simulink model "cq3_2019"  (R2024b)
settings: Solver=FixedStepAuto  StartTime=0.0  StopTime=10  FixedStep=0.001  RelTol=1e-3
libraries: simulink x3, Solver_SF x1
settings Model: SnapshotBufferSize=2  SnapshotInterval=1  Creator=user  LastModifiedBy=user

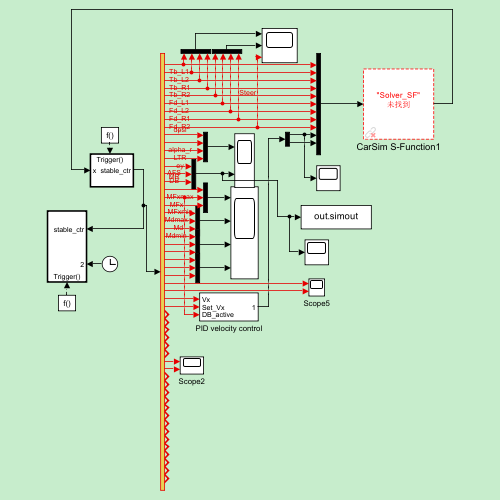
[thumbnail: Simulink's stored preview of the top-level diagram]
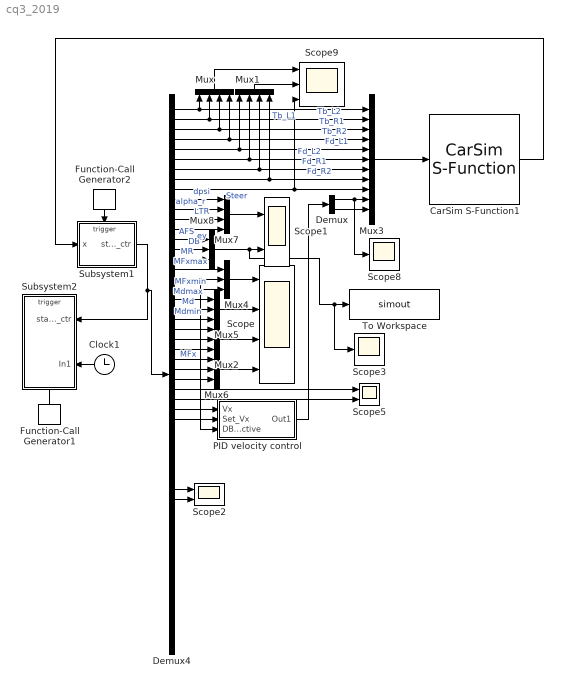
== system cq3_2019 ==
  CarSim S-Function1 : Solver_SF/CarSim S-Function  Priority=1  SIMFILE=simfile.sim
  Clock1 : Clock
  Demux : Demux  Outputs=2
  Demux4 : Demux  Outputs=54
  Function-Call Generator1 : simulink/Ports & Subsystems/Function-Call Generator  sample_time=0.01  numberOfIterations=1  DisallowWideOutput=off
  Function-Call Generator2 : simulink/Ports & Subsystems/Function-Call Generator  sample_time=0.01  numberOfIterations=1  DisallowWideOutput=off
  Mux : Mux
  Mux1 : Mux
  Mux{2,4..6,8} (5 alike) : Mux  Inputs=3
  Mux3 : Mux  Inputs=11
  Mux7 : Mux
  PID velocity control : Subsystem
  Scope : Scope  NumInputPorts=4
  Scope1 : Scope  NumInputPorts=2
  Scope2 : Scope  NumInputPorts=2
  Scope3 : Scope
  Scope5 : Scope  NumInputPorts=2
  Scope8 : Scope
  Scope9 : Scope  NumInputPorts=3
  Subsystem1 : Subsystem
  Subsystem2 : Subsystem
  To Workspace : ToWorkspace  VariableName=simout  SaveFormat=Timeseries  SampleTime=-1
  wires:
  Demux4/4 -> Mux/4, Mux3/4  "Tb_R2"
  Demux4/19 -> Mux4/3  "MFxmin"
  Demux4/26 -> Mux6/1
  Demux4/21 -> Mux5/2  "Md"
  CarSim S-Function1/1 -> Subsystem1/1(x)
  Demux4/3 -> Mux/3, Mux3/3  "Tb_R1"
  Demux4/17 -> Mux4/1  "MFxmax"
  Demux4/18 -> Mux4/2, PID velocity control/3(DB_active)  "MFx"
  Demux4/8 -> Mux1/4, Mux3/8  "Fd_R2"
  Demux4/5 -> Mux1/1, Mux3/5  "Fd_L1"
  Demux4/15 -> Mux8/2  "DB"
  Demux4/27 -> Mux6/2
  Demux4/11 -> Mux7/2  "alpha_r"
  Demux4/20 -> Mux5/1  "Mdmax"
  Demux4/12 -> Mux7/3  "LTR"
  Demux4/10 -> Mux7/1  "dpsi"
  Demux4/9 -> Scope9/3, Mux3/9  "Steer"
  Demux4/14 -> Mux8/1  "AFS"
  Demux4/24 -> Mux2/2
  Demux4/6 -> Mux1/2, Mux3/6  "Fd_L2"
  Demux4/1 -> Mux/1, Mux3/1  "Tb_L1"
  Demux4/16 -> Mux8/3  "MR"
  Demux4/25 -> Mux2/3
  Demux4/22 -> Mux5/3  "Mdmin"
  Demux4/2 -> Mux/2, Mux3/2  "Tb_L2"
  Demux4/29 -> Scope5/1
  Demux4/23 -> Mux2/1
  Demux4/7 -> Mux1/3, Mux3/7  "Fd_R1"
  Function-Call Generator2/1 -> Subsystem1/Trigger
  Demux4/13 -> Mux7/4  "ey"
  Demux4/28 -> Mux6/3
  Demux/1 -> Scope8/1, Mux3/10
  Demux/2 -> Mux3/11
  Mux/1 -> Scope9/1
  Mux1/1 -> Scope9/2
  Mux4/1 -> Scope/1
  Mux5/1 -> Scope/2
  Mux2/1 -> Scope/3
  Mux6/1 -> Scope/4
  PID velocity control/1(Out1) -> Demux/1
  Mux7/1 -> Scope1/1
  Mux8/1 -> Scope3/1, To Workspace/1, Scope1/2
  Clock1/1 -> Subsystem2/2(In1)
  Subsystem1/1(stable_ctr) -> Subsystem2/1(stable_ctr), Demux4/1
  Function-Call Generator1/1 -> Subsystem2/Trigger
  Demux4/31 -> PID velocity control/1(Vx)
  Demux4/32 -> PID velocity control/2(Set_Vx)
  Demux4/39 -> Scope2/1
  Demux4/40 -> Scope2/2
  Mux3/1 -> CarSim S-Function1/1
  Demux4/30 -> Scope5/2

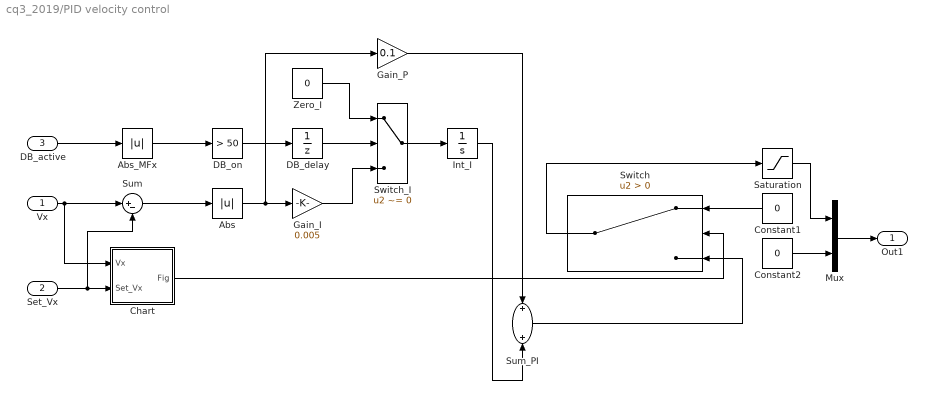
== system cq3_2019/PID velocity control ==
  Vx : Inport
  Set_Vx : Inport  Port=2
  DB_active : Inport  Port=3
  Abs : Abs  SaturateOnIntegerOverflow=off
  Abs_MFx : Abs  SaturateOnIntegerOverflow=off
  Chart : Stateflow chart  TreatAsAtomicUnit=on
  Constant1 : Constant  Value=0
  Constant2 : Constant  Value=0
  DB_delay : UnitDelay  SampleTime=-1  HasFrameUpgradeWarning=on
  DB_on : simulink/Logic and Bit Operations/Compare To Constant  relop=>  const=50  OutDataTypeStr=uint8
  Gain_I : Gain  Gain=0.005
  Gain_P : Gain  Gain=0.1
  Int_I : Integrator
  Mux : Mux  Inputs=2
  Saturation : Saturate  UpperLimit=1  LowerLimit=0
  Sum : Sum  Inputs=|+-
  Sum_PI : Sum
  Switch : Switch  Criteria=u2 > Threshold  SaturateOnIntegerOverflow=off  InputSameDT=off
  Switch_I : Switch  Criteria=u2 ~= 0  SaturateOnIntegerOverflow=off  InputSameDT=off
  Zero_I : Constant  Value=0
  Out1 : Outport
  wires:
  Chart/1(Fig) -> Switch/2
  Set_Vx/1 -> Sum/2, Chart/2(Set_Vx)
  DB_active/1 -> Abs_MFx/1
  DB_delay/1 -> Switch_I/2
  Vx/1 -> Chart/1(Vx), Sum/1
  DB_on/1 -> DB_delay/1
  Abs_MFx/1 -> DB_on/1
  Saturation/1 -> Mux/1
  Sum/1 -> Abs/1
  Abs/1 -> Gain_P/1, Gain_I/1
  Zero_I/1 -> Switch_I/1
  Gain_I/1 -> Switch_I/3
  Constant1/1 -> Switch/1
  Gain_P/1 -> Sum_PI/1
  Switch_I/1 -> Int_I/1
  Int_I/1 -> Sum_PI/2
  Sum_PI/1 -> Switch/3
  Switch/1 -> Saturation/1
  Constant2/1 -> Mux/2
  Mux/1 -> Out1/1

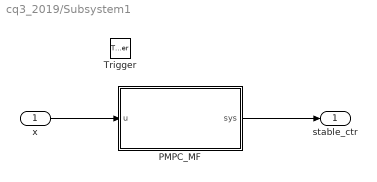
== system cq3_2019/Subsystem1 ==
  x : Inport
  Trigger : TriggerPort  TriggerType=function-call  VariantControl=(inherit)  PortDimensions=1
  PMPC_MF : MATLAB Function  TreatAsAtomicUnit=on
  stable_ctr : Outport
  wires:
  PMPC_MF/1(sys) -> stable_ctr/1
  x/1 -> PMPC_MF/1(u)

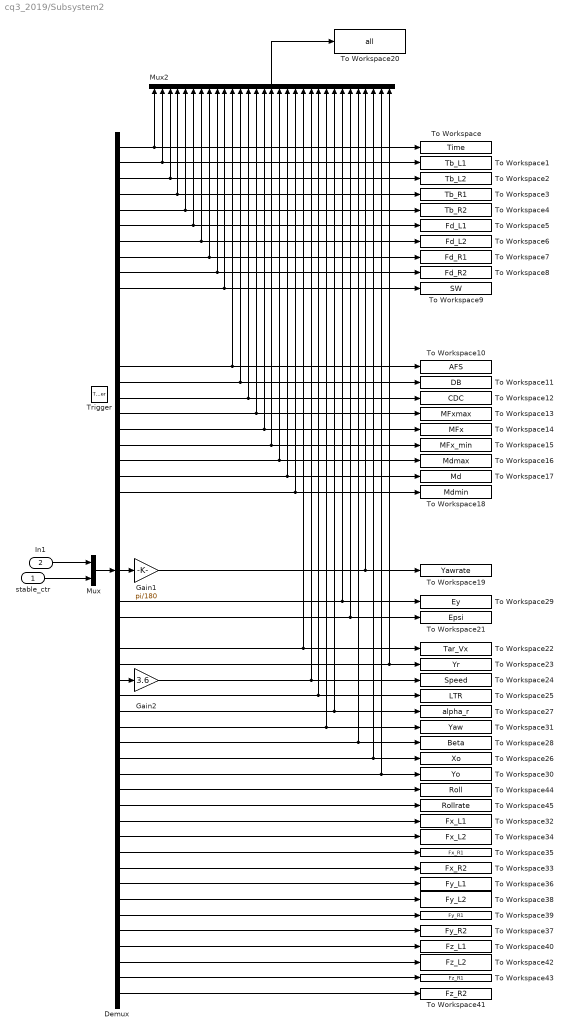
== system cq3_2019/Subsystem2 ==
  stable_ctr : Inport
  In1 : Inport  Port=2
  Trigger : TriggerPort  TriggerType=function-call  VariantControl=(inherit)  PortDimensions=1
  Demux : Demux  Outputs=55
  Gain1 : Gain  Gain=pi/180
  Gain2 : Gain  Gain=3.6
  Mux : Mux  Inputs=2
  Mux2 : Mux  Inputs=31
  To Workspace : ToWorkspace  VariableName=Time  SampleTime=-1
  To Workspace1 : ToWorkspace  VariableName=Tb_L1  SampleTime=-1
  To Workspace10 : ToWorkspace  VariableName=AFS  SampleTime=-1
  To Workspace11 : ToWorkspace  VariableName=DB  SampleTime=-1
  To Workspace12 : ToWorkspace  VariableName=CDC  SampleTime=-1
  To Workspace13 : ToWorkspace  VariableName=MFxmax  SampleTime=-1
  To Workspace14 : ToWorkspace  VariableName=MFx  SampleTime=-1
  To Workspace15 : ToWorkspace  VariableName=MFx_min  SampleTime=-1
  To Workspace16 : ToWorkspace  VariableName=Mdmax  SampleTime=-1
  To Workspace17 : ToWorkspace  VariableName=Md  SampleTime=-1
  To Workspace18 : ToWorkspace  VariableName=Mdmin  SampleTime=-1
  To Workspace19 : ToWorkspace  VariableName=Yawrate  SampleTime=-1
  To Workspace2 : ToWorkspace  VariableName=Tb_L2  SampleTime=-1
  To Workspace20 : ToWorkspace  VariableName=all  SampleTime=-1
  To Workspace21 : ToWorkspace  VariableName=Epsi  SampleTime=-1
  To Workspace22 : ToWorkspace  VariableName=Tar_Vx  SampleTime=-1
  To Workspace23 : ToWorkspace  VariableName=Yr  SampleTime=-1
  To Workspace24 : ToWorkspace  VariableName=Speed  SampleTime=-1
  To Workspace25 : ToWorkspace  VariableName=LTR  SampleTime=-1
  To Workspace26 : ToWorkspace  VariableName=Xo  SampleTime=-1
  To Workspace27 : ToWorkspace  VariableName=alpha_r  SampleTime=-1
  To Workspace28 : ToWorkspace  VariableName=Beta  SampleTime=-1
  To Workspace29 : ToWorkspace  VariableName=Ey  SampleTime=-1
  To Workspace3 : ToWorkspace  VariableName=Tb_R1  SampleTime=-1
  To Workspace30 : ToWorkspace  VariableName=Yo  SampleTime=-1
  To Workspace31 : ToWorkspace  VariableName=Yaw  SampleTime=-1
  To Workspace32 : ToWorkspace  VariableName=Fx_L1  SampleTime=-1
  To Workspace33 : ToWorkspace  VariableName=Fx_R2  SampleTime=-1
  To Workspace34 : ToWorkspace  VariableName=Fx_L2  SampleTime=-1
  To Workspace35 : ToWorkspace  VariableName=Fx_R1  SampleTime=-1
  To Workspace36 : ToWorkspace  VariableName=Fy_L1  SampleTime=-1
  To Workspace37 : ToWorkspace  VariableName=Fy_R2  SampleTime=-1
  To Workspace38 : ToWorkspace  VariableName=Fy_L2  SampleTime=-1
  To Workspace39 : ToWorkspace  VariableName=Fy_R1  SampleTime=-1
  To Workspace4 : ToWorkspace  VariableName=Tb_R2  SampleTime=-1
  To Workspace40 : ToWorkspace  VariableName=Fz_L1  SampleTime=-1
  To Workspace41 : ToWorkspace  VariableName=Fz_R2  SampleTime=-1
  To Workspace42 : ToWorkspace  VariableName=Fz_L2  SampleTime=-1
  To Workspace43 : ToWorkspace  VariableName=Fz_R1  SampleTime=-1
  To Workspace44 : ToWorkspace  VariableName=Roll  SampleTime=-1
  To Workspace45 : ToWorkspace  VariableName=Rollrate  SampleTime=-1
  To Workspace5 : ToWorkspace  VariableName=Fd_L1  SampleTime=-1
  To Workspace6 : ToWorkspace  VariableName=Fd_L2  SampleTime=-1
  To Workspace7 : ToWorkspace  VariableName=Fd_R1  SampleTime=-1
  To Workspace8 : ToWorkspace  VariableName=Fd_R2  SampleTime=-1
  To Workspace9 : ToWorkspace  VariableName=SW  SampleTime=-1
  wires:
  Mux/1 -> Demux/1
  stable_ctr/1 -> Mux/2
  In1/1 -> Mux/1
  Demux/1 -> To Workspace/1, Mux2/1
  Demux/2 -> Mux2/2, To Workspace1/1
  Demux/3 -> To Workspace2/1, Mux2/3
  Demux/4 -> Mux2/4, To Workspace3/1
  Demux/5 -> Mux2/5, To Workspace4/1
  Demux/6 -> Mux2/6, To Workspace5/1
  Demux/7 -> To Workspace6/1, Mux2/7
  Demux/8 -> Mux2/8, To Workspace7/1
  Demux/9 -> Mux2/9, To Workspace8/1
  Demux/10 -> Mux2/10, To Workspace9/1
  Demux/15 -> Mux2/11, To Workspace10/1
  Demux/16 -> Mux2/12, To Workspace11/1
  Demux/17 -> Mux2/13, To Workspace12/1
  Demux/18 -> Mux2/14, To Workspace13/1
  Demux/19 -> To Workspace14/1, Mux2/15
  Demux/20 -> Mux2/16, To Workspace15/1
  Demux/21 -> Mux2/17, To Workspace16/1
  Demux/22 -> Mux2/18, To Workspace17/1
  Demux/23 -> Mux2/19, To Workspace18/1
  Demux/28 -> Gain1/1
  Demux/31 -> Mux2/26, To Workspace21/1
  Demux/34 -> Mux2/31, To Workspace23/1
  Demux/35 -> Gain2/1
  Demux/37 -> Mux2/24, To Workspace27/1
  Mux2/1 -> To Workspace20/1
  Gain1/1 -> To Workspace19/1, Mux2/28
  Demux/30 -> Mux2/25, To Workspace29/1
  Gain2/1 -> Mux2/21, To Workspace24/1
  Demux/36 -> Mux2/22, To Workspace25/1
  Demux/38 -> Mux2/23, To Workspace31/1
  Demux/39 -> Mux2/27, To Workspace28/1
  Demux/40 -> Mux2/29, To Workspace26/1
  Demux/41 -> Mux2/30, To Workspace30/1
  Demux/33 -> Mux2/20, To Workspace22/1
  Demux/47 -> To Workspace33/1
  Demux/52 -> To Workspace40/1
  Demux/44 -> To Workspace32/1
  Demux/53 -> To Workspace42/1
  Demux/49 -> To Workspace38/1
  Demux/46 -> To Workspace35/1
  Demux/50 -> To Workspace39/1
  Demux/51 -> To Workspace37/1
  Demux/54 -> To Workspace43/1
  Demux/45 -> To Workspace34/1
  Demux/55 -> To Workspace41/1
  Demux/42 -> To Workspace44/1
  Demux/48 -> To Workspace36/1
  Demux/43 -> To Workspace45/1

== matlab function cq3_2019/Subsystem1/PMPC_MF ==
  data: u input; sys output; PMPC_P parameter
function sys = pmpc_block_blk(u, PMPC_P)
%#codegen
%  块里只写一行调用 —— 实体在 pmpc_block.m,
%  这样可以单独对它跑 codegen 调试(见 cg_block.m)。
sys = pmpc_block(u, PMPC_P);
end

== stateflow chart cq3_2019/PID velocity control/Chart ==
  (default) -> (junction 4)
  (junction 4) -> (junction 7) [order 2] : [Vx>=Set_Vx]
  (junction 4) -> (junction 6) [order 1] : [Vx<Set_Vx]{Fig=-1;}
  (junction 7) -> (junction 11)
  (junction 11) -> (junction 13) [order 1] : [Vx>Set_Vx]{Fig=1;}
  (junction 11) -> (junction 15) [order 2] : [Vx==Set_Vx]{Fig=0;}
  (junction 13) -> (junction 17)
  (junction 15) -> (junction 6)
  (junction 17) -> (junction 15)
  data: Vx input double; Set_Vx input double; Fig output
